simulink model "M5_motor_load_gearbox_friction_rated_gravity"  (Simulink 10.2)
settings: Solver=ode4  StartTime=0.0  StopTime=4  FixedStep=T_s*0.1  RelTol=1e-3
undefined symbols (not defined in the file): b_eq, g, i_rated, J_eq, k, L, L_l, m_l, N_opt, R, tau_c, tau_m_rated, theta_0
libraries: simulink x1
settings Model: Creator=ioannis  LastModifiedBy=mfocchi
settings DataIOCC: SaveFormat=Dataset  SignalLoggingSaveFormat=Dataset
settings OptimizationCC: LifeSpan=auto
settings DebuggingCC: UnderspecifiedInitializationDetection=Simplified  MergeDetectMultiDrivingBlocksExec=error  FcnCallInpInsideContextMsg=error  SFUnexpectedBacktrackingDiag=error  SFNoUnconditionalDefaultTransitionDiag=error  SFExecutionAtInitializationDiag=warning
settings HardwareCC: ProdBitPerPointer=64  ProdBitPerSizeT=64  ProdBitPerPtrDiffT=64  ProdLargestAtomicFloat=Float  ProdIntDivRoundTo=Zero  ProdEndianess=LittleEndian  ProdWordSize=64  ProdHWDeviceType=Intel->x86-64 (Windows64)
settings ModelReferenceCC: PropagateSignalLabelsOutOfModel=on
settings SFSimCC: SimUseLocalCustomCode=on
settings RTWCC: RTWUseLocalCustomCode=on
settings CodeAppCC: StateflowObjectComments=off
settings GRTTargetCC: TargetLangStandard=C99 (ISO)  CombineOutputUpdateFcns=on  GRTInterface=off
settings ConfigComp: CovMetricSettings=dwe  CovSaveCumulativeToWorkspaceVar=off  CovSaveSingleToWorkspaceVar=off  CovExternalEMLEnable=on

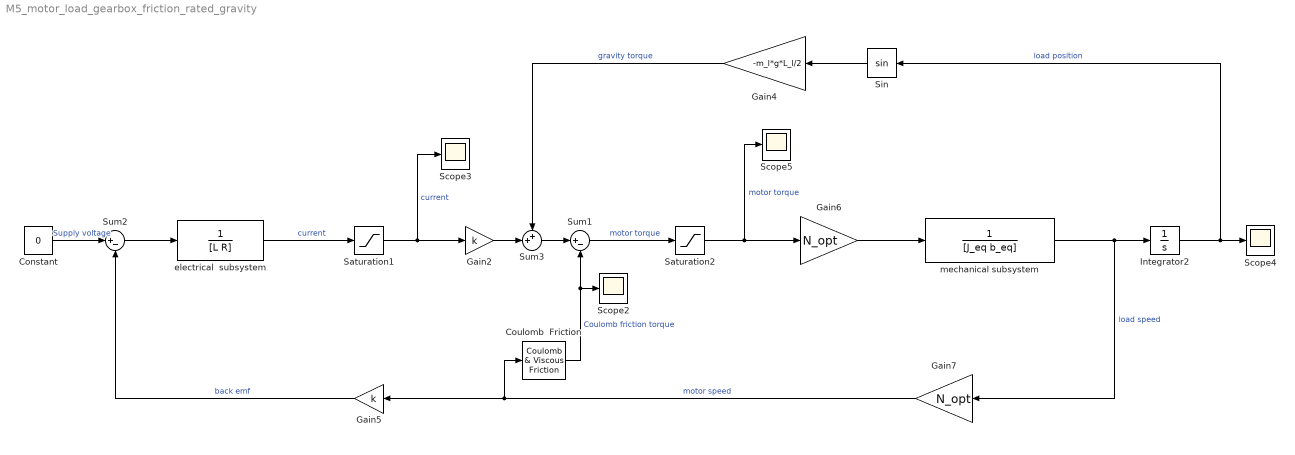
== system M5_motor_load_gearbox_friction_rated_gravity ==
  Constant : Constant  Value=0
  Coulomb  Friction : simulink/Discontinuities/Coulomb & Viscous Friction  offset=tau_c*0  gain=0
  Gain2 : Gain  Gain=k
  Gain4 : Gain  Gain=-m_l*g*L_l/2
  Gain5 : Gain  Gain=k
  Gain6 : Gain  Gain=N_opt
  Gain7 : Gain  Gain=N_opt
  Integrator2 : Integrator  InitialCondition=theta_0
  Saturation1 : Saturate  UpperLimit=i_rated  LowerLimit=-i_rated
  Saturation2 : Saturate  UpperLimit=tau_m_rated  LowerLimit=-tau_m_rated
  Scope{2..5} (4 alike) : Scope
  Sin : Trigonometry
  Sum1 : Sum  Inputs=|+-
  Sum2 : Sum  Inputs=|+-
  Sum3 : Sum  Inputs=++|
  electrical  subsystem : TransferFcn  Denominator=[L R]
  mechanical subsystem : TransferFcn  Denominator=[J_eq b_eq]
  wires:
  Gain7/1 -> Coulomb  Friction/1, Gain5/1  "motor speed"
  Constant/1 -> Sum2/1  "Supply voltage"
  mechanical subsystem/1 -> Gain7/1, Integrator2/1  "load speed"
  Sum2/1 -> electrical  subsystem/1
  Coulomb  Friction/1 -> Sum1/2, Scope2/1  "Coulomb friction torque"
  electrical  subsystem/1 -> Saturation1/1  "current"
  Saturation1/1 -> Scope3/1, Gain2/1  "current"
  Sum1/1 -> Saturation2/1  "motor torque"
  Saturation2/1 -> Scope5/1, Gain6/1  "motor torque"
  Gain6/1 -> mechanical subsystem/1
  Integrator2/1 -> Sin/1, Scope4/1  "load position"
  Sin/1 -> Gain4/1
  Gain2/1 -> Sum3/2
  Sum3/1 -> Sum1/1
  Gain4/1 -> Sum3/1  "gravity torque"
  Gain5/1 -> Sum2/2  "back emf"
